simulink model "RAVM"  (R2021b)
settings: Solver=ode23tb  StartTime=0.0  StopTime=Ts  MaxStep=1e-5  RelTol=1e-3  AbsTol=1e-3  EnableMultiTasking=on
values from neighbouring files (symbols this model uses):
  C1 = 1e-6    (= 1e-06)    [Parameter_preparation.m]    (also in TF.m)
  C2 = 180e-6    (= 0.00018)    [Parameter_preparation.m]    (also in TF.m)
  C3 = 1e-6    (= 1e-06)    [Parameter_preparation.m]    (also in TF.m)
  C4 = 100e-6    (= 0.0001)    [Parameter_preparation.m]    (also in TF.m)
  fs = 1/T/2    (= 20000)    [Parameter_preparation.m]
  L1 = 1e-6    (= 1e-06)    [Parameter_preparation.m]    (also in TF.m)
  L2 = 1e-6    (= 1e-06)    [Parameter_preparation.m]    (also in TF.m)
  Leq = Lp + Ls/(n^2)    (= 8.021e-05)    [Parameter_preparation.m]
  LM = 2600e-6    (= 0.0026)    [Parameter_preparation.m]
  n = 1/1    (= 1)    [Parameter_preparation.m]    (also in TF.m)
  R1 = 0.143    [Parameter_preparation.m]    (also in TF.m = 0.68)
  R2 = 0.094    [Parameter_preparation.m]    (also in TF.m = 0.68)
  Req = Rp + 2*Rsw + (Rs + 2*Rsw)/(n^2)    (= 0.501)    [Parameter_preparation.m]    (also in TF.m = 1.417)
  RM = 4600    [Parameter_preparation.m]    (also in TF.m = 2000)
  Ro = 20    [Parameter_preparation.m]    (also in TF.m = 0.5)
  Tsw = 1 / Fsw    (= 5e-05)    [Parameter_preparation.m]
  Vin = 100    [Parameter_preparation.m]    (also in TF.m)
  Vo = 0    [Parameter_preparation.m]    (also in TF.m)
  Vout = 100    [Parameter_preparation.m]
libraries: slpidlib x1
settings Model: Creator=Kai  LastModifiedBy=Administrator
settings SolverCC: AutoScaleAbsTol=off  AlgebraicLoopSolver=TrustRegion
settings DataIOCC: FinalStateName=xFinal_avg  InitialState=xFinal_avg  SaveFormat=Array  SignalLoggingSaveFormat=ModelDataLogs  ReturnWorkspaceOutputs=off  TimeSaveName=tout_avg  OutputSaveName=yout_avg
settings OptimizationCC: ExpressionDepthLimit=2147483647  LifeSpan=inf
settings DebuggingCC: UnderspecifiedInitializationDetection=Classic  MergeDetectMultiDrivingBlocksExec=none  SolverPrmCheckMsg=warning  MultiTaskDSMMsg=warning  MultiTaskCondExecSysMsg=none  StateNameClashWarn=warning  SFUnexpectedBacktrackingDiag=warning  SFNoUnconditionalDefaultTransitionDiag=warning  SFExecutionAtInitializationDiag=none  SFMachineParentedDataDiag=warning  ArithmeticOperatorsInVariantConditions=warning
settings HardwareCC: ProdBitPerPointer=32  ProdBitPerSizeT=32  ProdBitPerPtrDiffT=32  ProdLargestAtomicFloat=None  ProdIntDivRoundTo=Undefined  ProdEndianess=Unspecified  ProdWordSize=32  ProdHWDeviceType=32-bit Generic
settings ModelReferenceCC: PropagateSignalLabelsOutOfModel=off
settings SFSimCC: SimUseLocalCustomCode=off  CustomCodeUndefinedFunction=UseInterfaceOnly
settings RTWCC: RTWUseLocalCustomCode=off
settings CodeAppCC: StateflowObjectComments=on
settings GRTTargetCC: TargetLangStandard=C89/C90 (ANSI)
settings ConfigComp: CovMetricSettings=dw  CovSaveCumulativeToWorkspaceVar=on  CovSaveSingleToWorkspaceVar=on  CovExternalEMLEnable=off

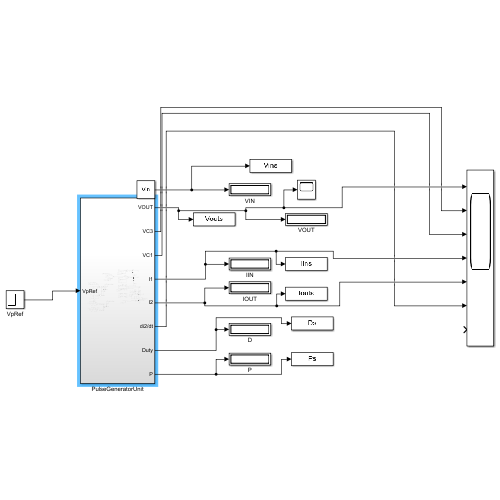
[thumbnail: Simulink's stored preview of the top-level diagram]
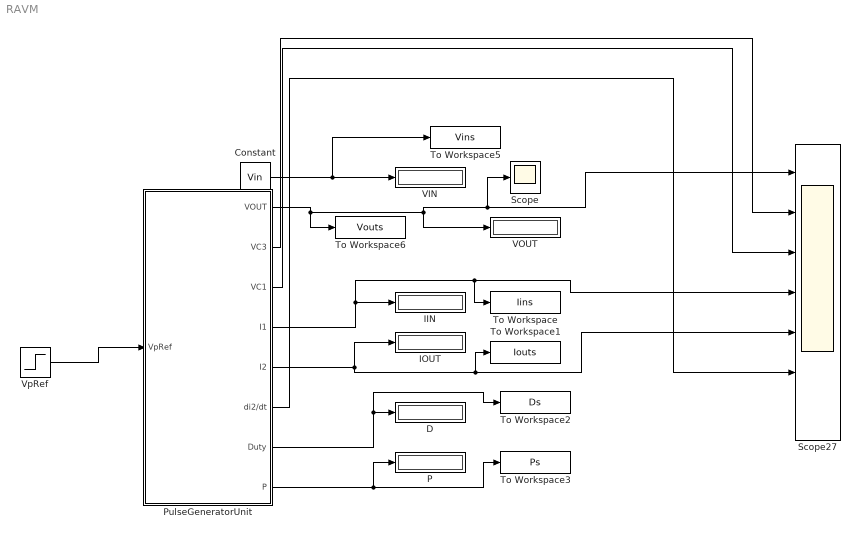
== system RAVM ==
  Constant : Constant  Value=Vin
  D : Display
  IIN : Display
  IOUT : Display
  P : Display
  PulseGeneratorUnit : Subsystem
  Scope : Scope
  Scope27 : Scope  NumInputPorts=7
  To Workspace : ToWorkspace  VariableName=Iins  SaveFormat=Timeseries  SampleTime=-1
      settings: Decimation=2
  To Workspace1 : ToWorkspace  VariableName=Iouts  SaveFormat=Timeseries  SampleTime=-1
      settings: Decimation=2
  To Workspace2 : ToWorkspace  VariableName=Ds  SaveFormat=Timeseries  SampleTime=-1
      settings: Decimation=2
  To Workspace3 : ToWorkspace  VariableName=Ps  SaveFormat=Timeseries  SampleTime=-1
      settings: Decimation=2
  To Workspace5 : ToWorkspace  VariableName=Vins  SaveFormat=Timeseries  SampleTime=-1
      settings: Decimation=2
  To Workspace6 : ToWorkspace  VariableName=Vouts  SaveFormat=Timeseries  SampleTime=-1
      settings: Decimation=2
  VIN : Display
  VOUT : Display
  VpRef : Step  Time=1/100000*10000/2  Before=Vout  After=Vout  SampleTime=0
  wires:
  VpRef/1 -> PulseGeneratorUnit/1(VpRef)
  PulseGeneratorUnit/1(VOUT) -> To Workspace6/1, Scope/1, Scope27/1, VOUT/1
  PulseGeneratorUnit/2(VC3) -> Scope27/2
  PulseGeneratorUnit/3(VC1) -> Scope27/3
  PulseGeneratorUnit/4(I1) -> To Workspace/1, Scope27/4, IIN/1
  PulseGeneratorUnit/5(I2) -> IOUT/1, To Workspace1/1, Scope27/5
  PulseGeneratorUnit/6(di2/dt) -> Scope27/6
  Constant/1 -> To Workspace5/1, VIN/1
  PulseGeneratorUnit/7(Duty) -> To Workspace2/1, D/1
  PulseGeneratorUnit/8(P) -> P/1, To Workspace3/1

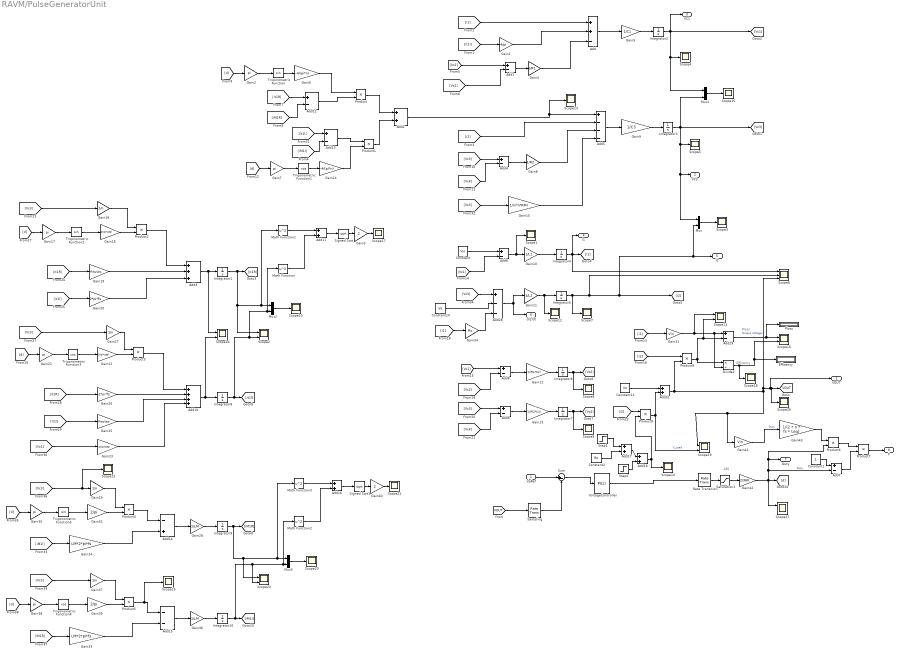
== system RAVM/PulseGeneratorUnit ==
  note: -180
  note: Efficency
  note: Ploss
  VpRef : Inport
  Add : Sum  Inputs=++-
  Add{1,4,6..9,12..13,29} (9 alike) : Sum  Inputs=+-
  Add10 : Sum  Inputs=++++
  Add{2,11,16..18,31} (6 alike) : Sum
  Add14 : Sum  Inputs=-+
  Add15 : Sum  Inputs=--
  Add28 : Sum  Inputs=+--
  Add3 : Sum  Inputs=+++
  Add5 : Sum  Inputs=+---
  Constant : Constant  Value=Vin
  Constant1 : Constant
  Constant10 : Constant  Value=Vo
  Constant11 : Constant  Value=Vo
  Constant2 : Constant  Value=Ro
  Divide2 : Product  Inputs=*/
  Efficency : Display
  Gain1 : Gain  Gain=4/pi
  Gain10 : Gain  Gain=1/L1
  Gain11 : Gain  Gain=1/L2
  Gain12 : Gain  Gain=1/(R1*C2)
  Gain13 : Gain  Gain=1/(R2*C4)
  Gain14 : Gain  Gain=-4/(pi*n)
  Gain15 : Gain  Gain=1/(n*n*RM)
  Gain{16,27,29,37} (4 alike) : Gain  Gain=1/n
  Gain{2,7,17,21,30,38} (6 alike) : Gain  Gain=pi
  Gain18 : Gain  Gain=2/(pi*Leq)
  Gain19 : Gain  Gain=-Req/Leq
  Gain20 : Gain  Gain=2*pi*fs
  Gain22 : Gain  Gain=2/(pi*Leq)
  Gain23 : Gain  Gain=-2/(pi*Leq)
  Gain24 : Gain  Gain=LM*2*pi*fs
  Gain25 : Gain  Gain=-Req/Leq
  Gain26 : Gain  Gain=-2*pi*fs
  Gain28 : Gain  Gain=1/LM
  Gain3 : Gain  Gain=2
  Gain31 : Gain  Gain=Vin
  Gain32 : Gain  Gain=2/pi
  Gain33 : Gain  Gain=LM*2*pi*fs
  Gain34 : Gain  Gain=Ro
  Gain36 : Gain  Gain=1/LM
  Gain39 : Gain  Gain=2/pi
  Gain4 : Gain  Gain=1/R1
  Gain40 : Gain  Gain=2
  Gain41 : Gain  Gain=Vin
  Gain42 : Gain  Gain=2/360
  Gain43 : Gain  Gain=1/(2 * n * fs * Leq)
  Gain5 : Gain  Gain=1/C1
  Gain6 : Gain  Gain=-4/(pi*n)
  Gain8 : Gain  Gain=1/R2
  Gain9 : Gain  Gain=1/C3
  Integrator{1,4..5,8..10} (6 alike) : Integrator
  Integrator2 : Integrator  InitialCondition=Vin
  Integrator3 : Integrator  InitialCondition=Vo
  Integrator6 : Integrator  InitialCondition=Vin
  Integrator7 : Integrator  InitialCondition=Vo
  Math Function{,1..3} (4 alike) : Math  Operator=square  SignedPower=on  SaturateOnIntegerOverflow=on
  Mux{,1..3} (4 alike) : Mux  Inputs=2
  Ploss : Display
  Product{,1..9} (10 alike) : Product  RndMeth=Zero
  Rate Transition : RateTransition
  Sampling : RateTransition
  Saturation1 : Saturate  UpperLimit=180  LowerLimit=-180
  Scope{1,3..5,7..10,12..15,17..18,20..21,23,25..26} (19 alike) : Scope
  Scope{2,11,16,19,22,24,27} (7 alike) : Scope  NumInputPorts=2
  Scope6 : Scope  NumInputPorts=3
  Signed Sqrt : Sqrt  SaturateOnIntegerOverflow=on
  Signed Sqrt1 : Sqrt  SaturateOnIntegerOverflow=on
  Step1 : Step  Time=0.2  After=-4  SampleTime=0
  Step2 : Step  Time=0.4  After=8  SampleTime=0
  Sum : Sum  Inputs=|+-
  Trigonometric Function : Trigonometry
  Trigonometric Function1 : Trigonometry  Operator=cos
  Trigonometric Function2 : Trigonometry
  Trigonometric Function3 : Trigonometry  Operator=cos
  Trigonometric Function4 : Trigonometry  Operator=cos
  Trigonometric Function5 : Trigonometry
  VoltageController : slpidlib/PID Controller  Controller=PI  Form=Parallel  TimeDomain=Discrete-time  UseExternalTs=off  SampleTime=Tsw  IntegratorMethod=Forward Euler  FilterMethod=Forward Euler  ControllerParametersSource=internal  P=0.033/2  I=46  D=0  UseFilter=on  N=100  TunerSelectOption=Transfer Function Based (PID Tuner App)  InitialConditionSource=internal  InitialConditionForIntegrator=0  InitialConditionForFilter=0  DifferentiatorICPrevScaledInput=0  ExternalReset=none  TrackingMode=off  Kt=1  LimitOutput=off  SatLimitsSource=internal  UpperSaturationLimit=inf  LowerSaturationLimit=-inf  LinearizeAsGain=on  AntiWindupMode=none  Kb=1  POutMin=[]  POutMax=[]  IOutMin=[]  IOutMax=[]  DOutMin=[]  DOutMax=[]  NOutMin=[]  NOutMax=[]  SumOutMin=[]  SumOutMax=[]  SaturationOutMin=[]  SaturationOutMax=[]  PParamMin=[]  PParamMax=[]  IParamMin=[]  IParamMax=[]  DParamMin=[]  DParamMax=[]  NParamMin=[]  NParamMax=[]  KbParamMin=[]  KbParamMax=[]  KtParamMin=[]  KtParamMax=[]  KbOutMin=[]  KbOutMax=[]  KtOutMin=[]  KtOutMax=[]  IntegratorOutMin=[]  IntegratorOutMax=[]  FilterOutMin=[]  FilterOutMax=[]  SumI1OutMin=[]  SumI1OutMax=[]  SumI2OutMin=[]  SumI2OutMax=[]  SumI3OutMin=[]  SumI3OutMax=[]  SumI4OutMin=[]  SumI4OutMax=[]  SumDOutMin=[]  SumDOutMax=[]  DifferentiatorOutMin=[]  DifferentiatorOutMax=[]  FilterDiffOutCoefMin=[]  FilterDiffOutCoefMax=[]  ReciprocalOutMin=[]  ReciprocalOutMax=[]  SumDenOutMin=[]  SumDenOutMax=[]  SumNumOutMin=[]  SumNumOutMax=[]  DivideOutMin=[]  DivideOutMax=[]  UdiffTsProdOutMin=[]  UdiffTsProdOutMax=[]  NTsProdOutMin=[]  NTsProdOutMax=[]  UintegralTsProdOutMin=[]  UintegralTsProdOutMax=[]  UngainTsProdOutMin=[]  UngainTsProdOutMax=[]  IntegratorContinuousStateAttributes=''  IntegratorStateMustResolveToSignalObject=off  IntegratorRTWStateStorageClass=Auto  FilterContinuousStateAttributes=''  FilterStateMustResolveToSignalObject=off  FilterRTWStateStorageClass=Auto  ParallelPVariant=InternalParameters  IdealPVariant=Disabled  IVariant=InternalParameters  DVariant=Disabled  IntegratorVariant=Discrete  SatVariant=Disabled  AWVariant=Passthrough  PCopyVariant=Disabled  TRVariant=Disabled  FdbkBlocksVariant=Forward  IdealPFdbkVariant=Disabled  SatFdbkVariant=Disabled  DerivativeFilterVariant=Disabled  NVariant=Disabled  NCopyVariant=Disabled_SignalSpec  FilterICVariant=Disabled  IntegratorICVariant=InternalICs  ExternalResetVariant=Disabled  TRSumVariant=Passthrough  SumFdbkVariant=Disabled  SumVariant=Sum_PI  TsampFilterVariant=InternalTs  TsampNgainVariant=Passthrough  TsampIntegralVariant=Passthrough  ExternalSaturationOutDataTypeStr=Inherit: Same as second input
  VOUT : Outport
  VC3 : Outport  Port=2
  VC1 : Outport  Port=3
  I1 : Outport  Port=4
  I2 : Outport  Port=5
  di2/dt : Outport  Port=6
  Duty : Outport  Port=7
  P : Outport  Port=8
  tag scope: VOUT=global
  wires:
  VpRef/1 -> Sum/1
  Add31/1 -> Product9/2, VOUT/1, Scope26/1, [VOUT], Scope6/3, Gain41/1, Scope19/1  "Output Voltage"
  Sum/1 -> VoltageController/1
  Product/1 -> Add2/1
  Gain30/1 -> Trigonometric Function5/1
  [iM1I] -> Add13/2
  [Vc3] -> Gain37/1
  [iM1R] -> Add12/2
  [Vc3] -> Gain27/1
  Signed Sqrt/1 -> Gain3/1
  [Vc3] -> Scope23/1, Gain29/1
  Gain40/1 -> Scope21/1
  Integrator4/1 -> I1/1, Scope6/1, [i1]
  Mux3/1 -> Scope20/1
  Product5/1 -> Scope25/1, Add15/1
  Gain32/1 -> Product4/2
  Integrator10/1 -> Scope22/2, Mux3/2, Math Function2/1, [iM1I]
  Math Function3/1 -> Add16/1
  Gain28/1 -> Integrator9/1
  [d] -> Gain38/1
  Gain24/1 -> Add14/2
  [iM1I] -> Gain24/1
  Gain39/1 -> Product5/2
  Gain23/1 -> Add10/4
  Trigonometric Function4/1 -> Gain39/1
  Add14/1 -> Gain28/1
  Product4/1 -> Add14/1
  Gain27/1 -> Product3/1
  [Vc2] -> Add8/2
  Gain37/1 -> Product5/1
  Math Function/1 -> Add11/2
  Gain15/1 -> Add5/4
  Mux2/1 -> Scope10/1
  Mux/1 -> Scope3/1
  Gain1/1 -> Add/2
  Add12/1 -> Product/2
  Gain18/1 -> Product2/2
  Gain26/1 -> Add10/2
  Gain5/1 -> Integrator2/1
  Mux1/1 -> Scope15/1
  Integrator6/1 -> Scope8/1, [Vc2]
  Gain4/1 -> Add/3
  Trigonometric Function5/1 -> Gain32/1
  [Vc1] -> Add6/2
  [d] -> Gain30/1
  Gain19/1 -> Add3/2
  Gain3/1 -> Scope17/1
  [it1I] -> Gain25/1
  Gain11/1 -> Scope12/1, Integrator5/1
  [Vc3] -> Add28/1
  Add13/1 -> Product1/1
  Gain22/1 -> Product3/2
  [it1R] -> Gain26/1
  [Vc1] -> Gain23/1
  Math Function1/1 -> Add11/1
  [Vc2] -> Add1/2
  Constant11/1 -> Add31/1
  Trigonometric Function3/1 -> Gain22/1
  [i2] -> Product8/1
  Gain21/1 -> Trigonometric Function3/1
  [d] -> Gain21/1
  [i2] -> Product9/1
  [i2] -> Add5/2
  Add9/1 -> Gain13/1
  Gain17/1 -> Trigonometric Function2/1
  Product2/1 -> Add3/1
  Add2/1 -> Scope13/1, Add5/1
  Math Function2/1 -> Add16/2
  Product1/1 -> Add2/2
  Gain14/1 -> Product1/2
  [it1R] -> Gain19/1
  [d] -> Gain7/1
  Gain20/1 -> Add3/3
  Add3/1 -> Scope24/1, Integrator1/1
  [d] -> Gain2/1
  Gain6/1 -> Product/1
  Trigonometric Function/1 -> Gain6/1
  Trigonometric Function1/1 -> Gain14/1
  [i1] -> Gain31/1
  Product9/1 -> Scope11/2, Add29/2, Divide2/1
  Divide2/1 -> Efficency/1, Scope16/2, Scope18/1
  Integrator9/1 -> Scope22/1, Mux3/1, Math Function3/1, [iM1R]
  Add29/1 -> Ploss/1, Scope16/1
  Add5/1 -> Gain9/1
  Gain34/1 -> Add28/3
  Constant10/1 -> Add28/2
  Integrator3/1 -> [Vc3], Mux1/2, Scope5/1, VC3/1, Mux/1
  [Vc1] -> Add8/1
  Gain10/1 -> Integrator4/1
  Trigonometric Function2/1 -> Gain18/1
  Integrator5/1 -> Scope6/2, I2/1, Mux/2, [i2], Scope7/1
  Gain7/1 -> Trigonometric Function1/1
  Integrator7/1 -> Scope9/1, [Vc4]
  Integrator2/1 -> [Vc1], VC1/1, Mux1/1, Scope4/1
  Add4/1 -> Gain8/1
  [it1I] -> Gain1/1
  [Vc4] -> Add9/2
  Add/1 -> Gain5/1
  Integrator1/1 -> Math Function1/1, Mux2/1, Scope2/1, [it1R]
  [Vc3] -> Add9/1
  Gain31/1 -> Scope11/1, Divide2/2, Add29/1
  [Vc3] -> Gain15/1
  Gain9/1 -> Integrator3/1
  Add1/1 -> Gain4/1
  Gain12/1 -> Integrator6/1
  Add6/1 -> Scope1/1, Gain10/1
  Add16/1 -> Signed Sqrt1/1
  Constant/1 -> Add6/1
  Integrator8/1 -> Math Function/1, Mux2/2, Scope2/2, [it1I]
  Gain25/1 -> Add10/3
  [Vc3] -> Add4/1
  [Vc3] -> Gain16/1
  Gain33/1 -> Add15/2
  Product3/1 -> Add10/1
  Add8/1 -> Gain12/1
  Add28/1 -> Gain11/1, di2/dt/1
  [i2] -> Gain34/1
  Gain16/1 -> Product2/1
  Gain13/1 -> Integrator7/1
  [it1I] -> Gain20/1
  [i1] -> Add/1
  [Vc4] -> Add4/2
  Gain36/1 -> Integrator10/1
  Gain2/1 -> Trigonometric Function/1
  Signed Sqrt1/1 -> Gain40/1
  Gain38/1 -> Trigonometric Function4/1
  [d] -> Gain17/1
  [it1I] -> Add13/1
  Add11/1 -> Signed Sqrt/1
  Product8/1 -> Add31/2, Scope19/2  "V_Load"
  Gain8/1 -> Add5/3
  Gain29/1 -> Product4/1
  [Vc1] -> Add1/1
  Add10/1 -> Scope24/2, Integrator8/1
  Saturation1/1 -> Gain42/1
  [it1R] -> Add12/1
  [iM1R] -> Gain33/1
  Add15/1 -> Gain36/1
  Sampling/1 -> Sum/2
  [VOUT] -> Sampling/1
  Rate Transition/1 -> Saturation1/1
  Gain42/1 -> Product6/2, Duty/1, Add7/2, Scope27/1, [d]  "Duty"
  Gain41/1 -> Gain43/1  "Duty"
  Gain43/1 -> Product6/1
  Product6/1 -> Product7/1
  Constant1/1 -> Add7/1
  Add7/1 -> Product7/2
  Product7/1 -> P/1
  VoltageController/1 -> Rate Transition/1
  Step1/1 -> Add17/1
  Constant2/1 -> Add17/2
  Step2/1 -> Add18/2
  Add18/1 -> Scope14/1, Product8/2
  Add17/1 -> Add18/1
